simulink model "MotorPosition"  (R2020b)
settings: Solver=ode15s  StartTime=0.0  StopTime=0.2  RelTol=1e-3
model workspace (MAT data in the model file):
  J = 3.2284e-06
  K = 0.0274
  L = 2.75e-06
  R = 4
  b = 3.5077e-06
settings Model: Creator=Pavan  LastModifiedBy=Pavan
settings DataIOCC: SaveOutput=off  SaveTime=off

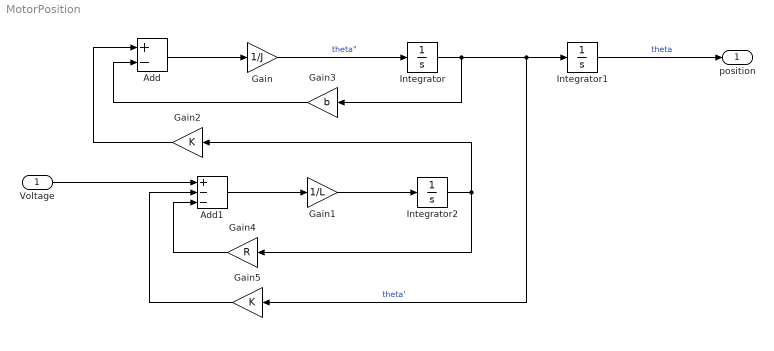
== system MotorPosition ==
  Voltage : Inport  OutDataTypeStr=double  PortDimensions=1
  Add : Sum  Inputs=+-
  Add1 : Sum  Inputs=+--
  Gain : Gain  Gain=1/J
  Gain1 : Gain  Gain=1/L
  Gain2 : Gain  Gain=K
  Gain3 : Gain  Gain=b
  Gain4 : Gain  Gain=R
  Gain5 : Gain  Gain=K
  Integrator : Integrator
  Integrator1 : Integrator
  Integrator2 : Integrator
  position : Outport  OutDataTypeStr=double  PortDimensions=1  SampleTime=0
  wires:
  Voltage/1 -> Add1/1
  Add/1 -> Gain/1
  Gain4/1 -> Add1/3
  Integrator1/1 -> position/1  "theta"
  Add1/1 -> Gain1/1
  Integrator/1 -> Gain3/1, Gain5/1, Integrator1/1  "theta'"
  Gain/1 -> Integrator/1  "theta\""
  Gain1/1 -> Integrator2/1
  Gain3/1 -> Add/2
  Gain2/1 -> Add/1
  Integrator2/1 -> Gain4/1, Gain2/1
  Gain5/1 -> Add1/2
